simulink model "Control_Systems_Drone_Sim"  (R2024b)
settings: Solver=VariableStepAuto  StartTime=0.0  StopTime=10  RelTol=1e-3
settings Model: Creator=HP  LastModifiedBy=ubuntu

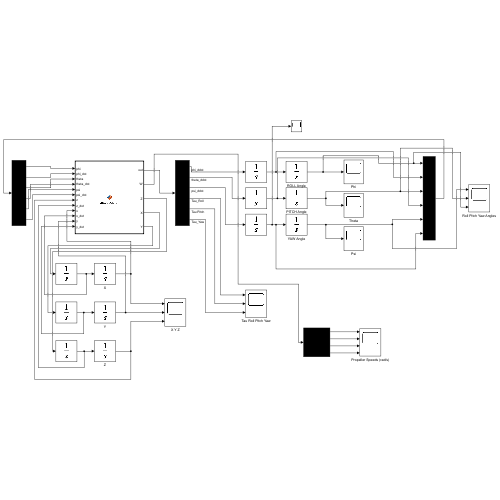
[thumbnail: Simulink's stored preview of the top-level diagram]
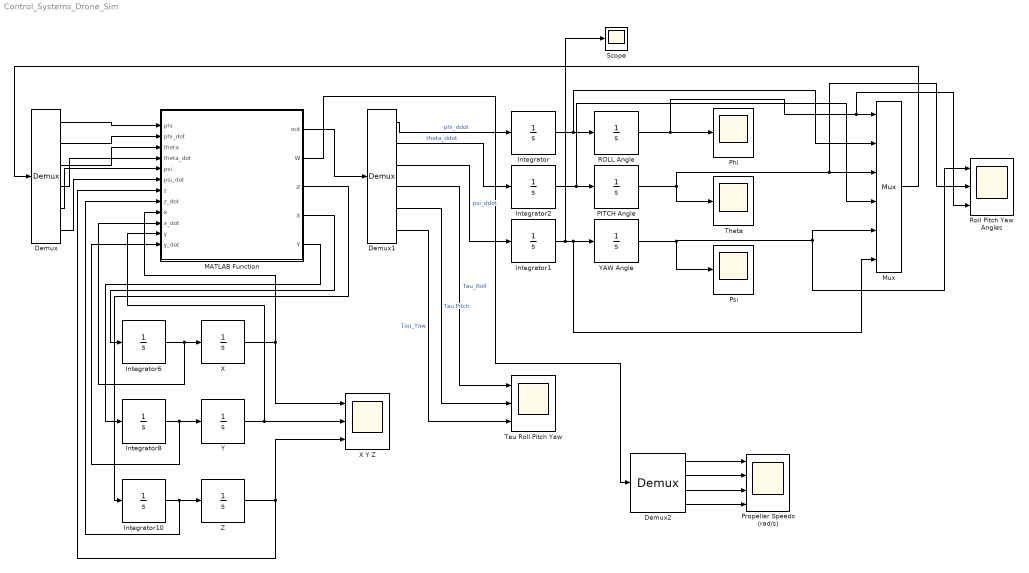
== system Control_Systems_Drone_Sim ==
  Demux : Demux  Outputs=6
  Demux1 : Demux  Outputs=6
  Demux2 : Demux
  Integrator{,1..2,6,8,10} (6 alike) : Integrator
  MATLAB Function : MATLAB Function  TreatAsAtomicUnit=on
  Mux : Mux  Inputs=6
  PITCH Angle : Integrator
  Phi : Scope
  Propeller Speeds (rad/s) : Scope  NumInputPorts=4
  Psi : Scope
  ROLL Angle : Integrator
  Roll Pitch Yaw Angles : Scope  NumInputPorts=3
  Scope : Scope
  Tau Roll Pitch Yaw : Scope  NumInputPorts=3
  Theta : Scope
  X : Integrator
  X Y Z : Scope  NumInputPorts=3
  Y : Integrator
  YAW Angle : Integrator
  Z : Integrator
  wires:
  Demux1/1 -> Integrator/1  "phi_ddot"
  Demux1/2 -> Integrator2/1  "theta_ddot"
  Demux1/3 -> Integrator1/1  "psi_ddot"
  Demux1/4 -> Tau Roll Pitch Yaw/1  "Tau_Roll"
  Demux1/5 -> Tau Roll Pitch Yaw/2  "Tau Pitch"
  Demux1/6 -> Tau Roll Pitch Yaw/3  "Tau_Yaw"
  Integrator2/1 -> Mux/4, PITCH Angle/1
  Integrator1/1 -> Scope/1, Mux/6, YAW Angle/1
  Integrator/1 -> Mux/2, ROLL Angle/1
  ROLL Angle/1 -> Roll Pitch Yaw Angles/3, Mux/1, Phi/1
  PITCH Angle/1 -> Roll Pitch Yaw Angles/2, Mux/3, Theta/1
  YAW Angle/1 -> Roll Pitch Yaw Angles/1, Mux/5, Psi/1
  Demux2/1 -> Propeller Speeds (rad/s)/1
  Demux2/2 -> Propeller Speeds (rad/s)/2
  Demux2/3 -> Propeller Speeds (rad/s)/3
  Demux2/4 -> Propeller Speeds (rad/s)/4
  Mux/1 -> Demux/1
  MATLAB Function/1(out) -> Demux1/1
  MATLAB Function/2(W) -> Demux2/1
  Integrator6/1 -> MATLAB Function/10(x_dot), X/1
  Integrator8/1 -> Y/1, MATLAB Function/12(y_dot)
  Integrator10/1 -> Z/1, MATLAB Function/8(z_dot)
  MATLAB Function/4(X) -> Integrator6/1
  MATLAB Function/5(Y) -> Integrator8/1
  MATLAB Function/3(Z) -> Integrator10/1
  X/1 -> MATLAB Function/9(x), X Y Z/1
  Y/1 -> MATLAB Function/11(y), X Y Z/2
  Z/1 -> X Y Z/3, MATLAB Function/7(z)
  Demux/1 -> MATLAB Function/1(phi)
  Demux/2 -> MATLAB Function/2(phi_dot)
  Demux/3 -> MATLAB Function/3(theta)
  Demux/4 -> MATLAB Function/4(theta_dot)
  Demux/5 -> MATLAB Function/5(psi)
  Demux/6 -> MATLAB Function/6(psi_dot)

== matlab function Control_Systems_Drone_Sim/MATLAB Function ==
  data: out output; W output; Z output; X output; Y output; phi input; phi_dot input; theta input; theta_dot input; psi input; psi_dot input; z input; z_dot input; x input; x_dot input; y input; y_dot input
function [out, W, Z, X, Y] = quadcopter(phi, phi_dot, theta, theta_dot, psi, psi_dot, z, z_dot, x, x_dot, y, y_dot)  

% Quadcopter Parameters (SI Units)
Ix = 4.856E-3;
Iy = 4.856E-3;
Iz = 8.801E-3;
m = 0.468;
l = 0.225;
g = 9.81;
k = 2.980E-6;
b = 1.140E-7;
Ax = 0.25;
Ay = 0.25;
Az = 0.25;

%%
% PD Control Gains
K_z_d = 2.5;
K_z_p = 1.5;
K_phi_d = 1.75;
K_theta_d = 1.75;
K_psi_d = 1.75;
K_phi_p = 6;
K_theta_p = 6;
K_psi_p = 6;

% Roll, Pitch and Yaw Position and Rate Commands
phi_dot_com = 0; %this is about x axis ... goes to -y
theta_dot_com = 0; %this is about y axis ... goes to +x
psi_dot_com = 0;
z_dot_com = 0;
phi_com = 0.0;
theta_com = 0.0;
psi_com = 0;
z_com = 2;

%%
% Roll, Pitch, and Yaw Torques
tau_phi = Ix*(K_phi_d*(phi_dot_com - phi_dot) + K_phi_p*(phi_com - phi));
tau_theta = Iy*(K_theta_d*(theta_dot_com - theta_dot) + K_theta_p*(theta_com - theta));
tau_psi = Iz*(K_psi_d*(psi_dot_com - psi_dot) + K_psi_p*(psi_com - psi));

T = (g + K_z_d*(z_dot_com - z_dot) + K_z_p*(z_com - z)) * (m / (cos(phi)*cos(theta)));
w1 = ((T/(4*k)) - tau_theta/(2*k*l) - tau_psi/(4*b))^0.5;
w2 = ((T/(4*k)) - tau_phi/(2*k*l) + tau_psi/(4*b))^0.5;
w3 = ((T/(4*k)) + tau_theta/(2*k*l) - tau_psi/(4*b))^0.5;
w4 = ((T/(4*k)) + tau_phi/(2*k*l) + tau_psi/(4*b))^0.5;

% eta =[phi theta psi]'
% J*eta_ddot + C*eta_dot = [tau_phi tau_theta tau_psi]'

J = zeros(3,3);
C = zeros(3,3);

%J Matrix
J(1,1) = Ix;
J(1,2) = 0;
J(1,3) = -Ix*sin(theta);
J(2,1) = 0;
J(2,2) = Iy*(cos(phi))^2 + Iz*(sin(phi))^2;
J(2,3) = (Iy - Iz)*cos(phi)*sin(phi)*cos(theta);
J(3,1) = -Ix*sin(theta);
J(3,2) = (Iy - Iz)*cos(phi)*sin(phi)*cos(theta);
J(3,3) = Ix*(sin(theta))^2 + Iy*(sin(phi))^2*(cos(theta))^2 + Iz*(cos(phi))^2*(cos(theta))^2;


%C Matrix
C(1,1) = 0;
C(1,2) = (Iz - Iy)*(theta_dot*cos(phi)*sin(phi) + psi_dot*(sin(phi))^2*cos(theta)) + ...
         (Iz - Iy)*psi_dot*(cos(phi))^2*cos(theta) - Ix*psi_dot*cos(theta);
C(1,3) = (Iz - Iy)*psi_dot*cos(phi)*sin(phi)*(cos(theta))^2;

C(2,1) = (Iz - Iy)*(theta_dot*cos(phi)*sin(phi) + psi_dot*cos(phi)*cos(theta)) + ...
         (Iy - Iz)*psi_dot*(cos(phi))^2*cos(theta);
C(2,2) = (Iz - Iy)*phi_dot*cos(phi)*sin(phi);
C(2,3) = -Ix*psi_dot*sin(theta)*cos(theta) + Iy*psi_dot*(sin(phi))^2*sin(theta)*cos(theta) + ...
         Iz*psi_dot*(cos(phi))^2*sin(theta)*cos(theta);

C(3,1) = (Iy - Iz)*psi_dot*(cos(theta))^2*sin(phi)*cos(phi) - Ix*theta_dot*cos(theta);
C(3,2) = (Iz - Iy)*(theta_dot*cos(phi)*sin(phi) + phi_dot*(sin(phi))^2*cos(theta)) + ...
         (Iy - Iz)*phi_dot*(cos(phi))^2*cos(theta) + Ix*psi_dot*sin(theta)*cos(theta) - ...
         Iy*psi_dot*(sin(phi))^2*sin(theta)*cos(theta) - Iz*psi_dot*(cos(phi))^2*sin(theta)*cos(theta);
C(3,3) = (Iy - Iz)*phi_dot*cos(phi)*sin(phi)*(cos(theta))^2 - Iy*theta_dot*(sin(phi))^2*cos(theta)*sin(theta) - ...
         Iz*theta_dot*(cos(phi))^2*cos(theta)*sin(theta) + Ix*theta_dot*cos(theta)*sin(theta);

B = [tau_phi tau_theta tau_psi]';

N = [phi_dot theta_dot psi_dot]';

W = [w1 w2 w3 w4]';

z_ddot = (T/m)*(cos(phi)*cos(theta)) - g - (Az/m)*z_dot;
x_ddot = (T/m)*(sin(phi)*sin(theta)*cos(psi) + cos(phi)*sin(psi)) - (Ax/m)*x_dot;
y_ddot = (T/m)*(-sin(phi)*cos(psi) + cos(phi)*sin(theta)*sin(psi)) - (Ay/m)*y_dot;

X = x_ddot;
Y = y_ddot;
Z = z_ddot;
out = [inv(J)*(B-C*N); B];
end
